simulink model "VikTask2"  (Simulink 7.8)
settings: Solver=ode45  StartTime=0.0  StopTime=10.0  RelTol=1e-3
libraries: simulink x3
settings Model: Creator=--  LastModifiedBy=--

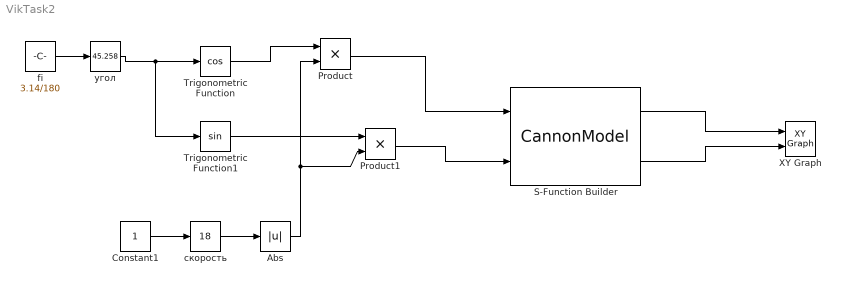
== system VikTask2 ==
  Abs : Abs
  Constant1 : Constant
  Product : Product  RndMeth=Zero
  Product1 : Product  RndMeth=Zero
  S-Function Builder : S-Function  InitFcn=try, set_param(gcb,'FunctionName',''), end  FunctionName=CannonModel  Parameters=0.5,9.81  WizardData=DataTag0  EnableBusSupport=off  mask(S-Function Builder){}
      mask help: Simulink:masks:SFunctionBuilder_MD
      mask init:
      | val = [[.9  0.75 0.75 1 1 .9 .9 1]',[1 1 0.75 0.75 .9 .9 1 .9]'];try , sys = get_param(gcb,'SfunBuilderFcnName');if isempty(sys), sys = get_param(gcb,'FunctionName'); end,catch, sys = get_param(gcb,'FunctionName'); end
      settings: CopyFcn=set_param(gcbh,'LinkStatus','none')  PreSaveFcn=try, set_param(gcb,'FunctionName','CannonModel'), end  OpenFcn=sfunctionwizard(gcbh)
      mask Display: plot(val(:,1),val(:,2)),disp(sys), port_label('input',1,'u0'), port_label('input',2,'u1'), port_label('output',1,'y0'), port_label('output',2,'y1')
  Trigonometric Function : Trigonometry  Operator=cos
  Trigonometric Function1 : Trigonometry
  XY Graph : simulink/Sinks/XY Graph  xmin=0  xmax=100  ymin=0  ymax=30  st=-1
  fi : Constant  Value=3.14/180
  скорость : simulink/Math Operations/Slider Gain  low=0  gain=18  high=100
  угол : simulink/Math Operations/Slider Gain  low=0  gain=45.258  high=90
  wires:
  fi/1 -> угол/1
  угол/1 -> Trigonometric Function/1, Trigonometric Function1/1
  Constant1/1 -> скорость/1
  скорость/1 -> Abs/1
  Trigonometric Function/1 -> Product/1
  Abs/1 -> Product/2, Product1/2
  Trigonometric Function1/1 -> Product1/1
  Product/1 -> S-Function Builder/1
  Product1/1 -> S-Function Builder/2
  S-Function Builder/1 -> XY Graph/1
  S-Function Builder/2 -> XY Graph/2
